simulink model "model_aggressive"  (R2021a)
settings: Solver=VariableStepAuto  StartTime=0.0  StopTime=ToA(end)  RelTol=1e-3
values from neighbouring files (symbols this model uses):
  I = [Jx Jxy Jxz ... (first row only)    [init.m]
  m = 1.5    [init.m]
  pos_ref = [ pos_refx' pos_refy' pos_refz' ]    [trajplann3.m]
  t_ref = []    [trajplann3.m]
  vel_ref = [ vel_refx, vel_refy, vel_refz ]    [trajplann3.m]
undefined symbols (not defined in the file or in its folder): psi
libraries: pid_lib x6, vrlib x4, simulink x1
settings Model: Creator=iris  LastModifiedBy=iris

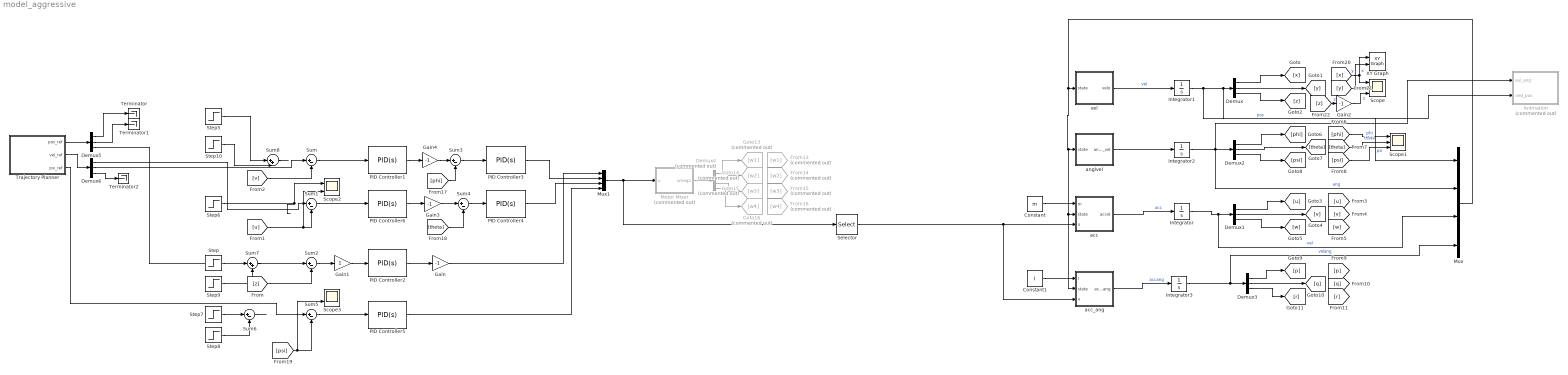
== system model_aggressive ==
  Animation : Subsystem  Commented=on
  Constant : Constant  Value=m
  Constant1 : Constant  Value=I
  Demux{,1..3,5..6} (6 alike) : Demux  Outputs=3
  Demux4 : Demux  Commented=on
  From13 : From  Commented=on  GotoTag=w1
  From14 : From  Commented=on  GotoTag=w2
  From15 : From  Commented=on  GotoTag=w3
  From16 : From  Commented=on  GotoTag=w4
  Gain{,2..4} (4 alike) : Gain  Gain=-1
  Gain1 : Gain
  Goto13 : Goto  Commented=on  GotoTag=w1
  Goto14 : Goto  Commented=on  GotoTag=w2
  Goto15 : Goto  Commented=on  GotoTag=w3
  Goto16 : Goto  Commented=on  GotoTag=w4
  Integrator{,1..3} (4 alike) : Integrator  InitialCondition=[0,0,0]
  Motor Mixer : MATLAB Function  Commented=on  TreatAsAtomicUnit=on
  Mux : Mux
  Mux1 : Mux
  PID Controller1 : pid_lib/PID Controller  Controller=PID  Form=Parallel  TimeDomain=Continuous-time  UseExternalTs=off  SampleTime=-1  IntegratorMethod=Forward Euler  FilterMethod=Forward Euler  ControllerParametersSource=internal  P=0.15  I=0  D=0.009  UseFilter=on  N=100  TunerSelectOption=Transfer Function Based (PID Tuner App)  InitialConditionSource=internal  InitialConditionForIntegrator=0  InitialConditionForFilter=0  DifferentiatorICPrevScaledInput=0  ExternalReset=none  TrackingMode=off  Kt=1  LimitOutput=off  SatLimitsSource=internal  UpperSaturationLimit=inf  LowerSaturationLimit=-inf  LinearizeAsGain=on  AntiWindupMode=none  Kb=1  POutMin=[]  POutMax=[]  IOutMin=[]  IOutMax=[]  DOutMin=[]  DOutMax=[]  NOutMin=[]  NOutMax=[]  SumOutMin=[]  SumOutMax=[]  SaturationOutMin=[]  SaturationOutMax=[]  PParamMin=[]  PParamMax=[]  IParamMin=[]  IParamMax=[]  DParamMin=[]  DParamMax=[]  NParamMin=[]  NParamMax=[]  KbParamMin=[]  KbParamMax=[]  KtParamMin=[]  KtParamMax=[]  KbOutMin=[]  KbOutMax=[]  KtOutMin=[]  KtOutMax=[]  IntegratorOutMin=[]  IntegratorOutMax=[]  FilterOutMin=[]  FilterOutMax=[]  SumI1OutMin=[]  SumI1OutMax=[]  SumI2OutMin=[]  SumI2OutMax=[]  SumI3OutMin=[]  SumI3OutMax=[]  SumI4OutMin=[]  SumI4OutMax=[]  SumDOutMin=[]  SumDOutMax=[]  DifferentiatorOutMin=[]  DifferentiatorOutMax=[]  FilterDiffOutCoefMin=[]  FilterDiffOutCoefMax=[]  ReciprocalOutMin=[]  ReciprocalOutMax=[]  SumDenOutMin=[]  SumDenOutMax=[]  SumNumOutMin=[]  SumNumOutMax=[]  DivideOutMin=[]  DivideOutMax=[]  UdiffTsProdOutMin=[]  UdiffTsProdOutMax=[]  NTsProdOutMin=[]  NTsProdOutMax=[]  UintegralTsProdOutMin=[]  UintegralTsProdOutMax=[]  UngainTsProdOutMin=[]  UngainTsProdOutMax=[]  IntegratorContinuousStateAttributes=''  IntegratorStateMustResolveToSignalObject=off  IntegratorRTWStateStorageClass=Auto  FilterContinuousStateAttributes=''  FilterStateMustResolveToSignalObject=off  FilterRTWStateStorageClass=Auto  ParallelPVariant=InternalParameters  IdealPVariant=Disabled  IVariant=InternalParameters  DVariant=InternalParameters  IntegratorVariant=Continuous  SatVariant=Disabled  AWVariant=Passthrough  PCopyVariant=Disabled  TRVariant=Disabled  FdbkBlocksVariant=Forward  IdealPFdbkVariant=Disabled  SatFdbkVariant=Disabled  DerivativeFilterVariant=ContFilter  NVariant=InternalParameters  NCopyVariant=Disabled  FilterICVariant=InternalICsFilter  IntegratorICVariant=InternalICs  ExternalResetVariant=Disabled  TRSumVariant=Passthrough  SumFdbkVariant=Disabled  SumVariant=Sum_PID  TsampFilterVariant=InternalTs  TsampNgainVariant=Passthrough  TsampIntegralVariant=Passthrough  ExternalSaturationOutDataTypeStr=Inherit: Same as second input
  PID Controller2 : pid_lib/PID Controller  Controller=PID  Form=Parallel  TimeDomain=Continuous-time  UseExternalTs=off  SampleTime=-1  IntegratorMethod=Forward Euler  FilterMethod=Forward Euler  ControllerParametersSource=internal  P=60  I=70  D=40  UseFilter=on  N=100  TunerSelectOption=Transfer Function Based (PID Tuner App)  InitialConditionSource=internal  InitialConditionForIntegrator=0  InitialConditionForFilter=0  DifferentiatorICPrevScaledInput=0  ExternalReset=none  TrackingMode=off  Kt=1  LimitOutput=off  SatLimitsSource=internal  UpperSaturationLimit=inf  LowerSaturationLimit=-inf  LinearizeAsGain=on  AntiWindupMode=none  Kb=1  POutMin=[]  POutMax=[]  IOutMin=[]  IOutMax=[]  DOutMin=[]  DOutMax=[]  NOutMin=[]  NOutMax=[]  SumOutMin=[]  SumOutMax=[]  SaturationOutMin=[]  SaturationOutMax=[]  PParamMin=[]  PParamMax=[]  IParamMin=[]  IParamMax=[]  DParamMin=[]  DParamMax=[]  NParamMin=[]  NParamMax=[]  KbParamMin=[]  KbParamMax=[]  KtParamMin=[]  KtParamMax=[]  KbOutMin=[]  KbOutMax=[]  KtOutMin=[]  KtOutMax=[]  IntegratorOutMin=[]  IntegratorOutMax=[]  FilterOutMin=[]  FilterOutMax=[]  SumI1OutMin=[]  SumI1OutMax=[]  SumI2OutMin=[]  SumI2OutMax=[]  SumI3OutMin=[]  SumI3OutMax=[]  SumI4OutMin=[]  SumI4OutMax=[]  SumDOutMin=[]  SumDOutMax=[]  DifferentiatorOutMin=[]  DifferentiatorOutMax=[]  FilterDiffOutCoefMin=[]  FilterDiffOutCoefMax=[]  ReciprocalOutMin=[]  ReciprocalOutMax=[]  SumDenOutMin=[]  SumDenOutMax=[]  SumNumOutMin=[]  SumNumOutMax=[]  DivideOutMin=[]  DivideOutMax=[]  UdiffTsProdOutMin=[]  UdiffTsProdOutMax=[]  NTsProdOutMin=[]  NTsProdOutMax=[]  UintegralTsProdOutMin=[]  UintegralTsProdOutMax=[]  UngainTsProdOutMin=[]  UngainTsProdOutMax=[]  IntegratorContinuousStateAttributes=''  IntegratorStateMustResolveToSignalObject=off  IntegratorRTWStateStorageClass=Auto  FilterContinuousStateAttributes=''  FilterStateMustResolveToSignalObject=off  FilterRTWStateStorageClass=Auto  ParallelPVariant=InternalParameters  IdealPVariant=Disabled  IVariant=InternalParameters  DVariant=InternalParameters  IntegratorVariant=Continuous  SatVariant=Disabled  AWVariant=Passthrough  PCopyVariant=Disabled  TRVariant=Disabled  FdbkBlocksVariant=Forward  IdealPFdbkVariant=Disabled  SatFdbkVariant=Disabled  DerivativeFilterVariant=ContFilter  NVariant=InternalParameters  NCopyVariant=Disabled  FilterICVariant=InternalICsFilter  IntegratorICVariant=InternalICs  ExternalResetVariant=Disabled  TRSumVariant=Passthrough  SumFdbkVariant=Disabled  SumVariant=Sum_PID  TsampFilterVariant=InternalTs  TsampNgainVariant=Passthrough  TsampIntegralVariant=Passthrough  ExternalSaturationOutDataTypeStr=Inherit: Same as second input
  PID Controller3 : pid_lib/PID Controller  Controller=PID  Form=Parallel  TimeDomain=Continuous-time  UseExternalTs=off  SampleTime=-1  IntegratorMethod=Forward Euler  FilterMethod=Forward Euler  ControllerParametersSource=internal  P=0.08  I=0.02  D=0.08  UseFilter=on  N=100  TunerSelectOption=Transfer Function Based (PID Tuner App)  InitialConditionSource=internal  InitialConditionForIntegrator=0  InitialConditionForFilter=0  DifferentiatorICPrevScaledInput=0  ExternalReset=none  TrackingMode=off  Kt=1  LimitOutput=off  SatLimitsSource=internal  UpperSaturationLimit=inf  LowerSaturationLimit=-inf  LinearizeAsGain=on  AntiWindupMode=none  Kb=1  POutMin=[]  POutMax=[]  IOutMin=[]  IOutMax=[]  DOutMin=[]  DOutMax=[]  NOutMin=[]  NOutMax=[]  SumOutMin=[]  SumOutMax=[]  SaturationOutMin=[]  SaturationOutMax=[]  PParamMin=[]  PParamMax=[]  IParamMin=[]  IParamMax=[]  DParamMin=[]  DParamMax=[]  NParamMin=[]  NParamMax=[]  KbParamMin=[]  KbParamMax=[]  KtParamMin=[]  KtParamMax=[]  KbOutMin=[]  KbOutMax=[]  KtOutMin=[]  KtOutMax=[]  IntegratorOutMin=[]  IntegratorOutMax=[]  FilterOutMin=[]  FilterOutMax=[]  SumI1OutMin=[]  SumI1OutMax=[]  SumI2OutMin=[]  SumI2OutMax=[]  SumI3OutMin=[]  SumI3OutMax=[]  SumI4OutMin=[]  SumI4OutMax=[]  SumDOutMin=[]  SumDOutMax=[]  DifferentiatorOutMin=[]  DifferentiatorOutMax=[]  FilterDiffOutCoefMin=[]  FilterDiffOutCoefMax=[]  ReciprocalOutMin=[]  ReciprocalOutMax=[]  SumDenOutMin=[]  SumDenOutMax=[]  SumNumOutMin=[]  SumNumOutMax=[]  DivideOutMin=[]  DivideOutMax=[]  UdiffTsProdOutMin=[]  UdiffTsProdOutMax=[]  NTsProdOutMin=[]  NTsProdOutMax=[]  UintegralTsProdOutMin=[]  UintegralTsProdOutMax=[]  UngainTsProdOutMin=[]  UngainTsProdOutMax=[]  IntegratorContinuousStateAttributes=''  IntegratorStateMustResolveToSignalObject=off  IntegratorRTWStateStorageClass=Auto  FilterContinuousStateAttributes=''  FilterStateMustResolveToSignalObject=off  FilterRTWStateStorageClass=Auto  ParallelPVariant=InternalParameters  IdealPVariant=Disabled  IVariant=InternalParameters  DVariant=InternalParameters  IntegratorVariant=Continuous  SatVariant=Disabled  AWVariant=Passthrough  PCopyVariant=Disabled  TRVariant=Disabled  FdbkBlocksVariant=Forward  IdealPFdbkVariant=Disabled  SatFdbkVariant=Disabled  DerivativeFilterVariant=ContFilter  NVariant=InternalParameters  NCopyVariant=Disabled  FilterICVariant=InternalICsFilter  IntegratorICVariant=InternalICs  ExternalResetVariant=Disabled  TRSumVariant=Passthrough  SumFdbkVariant=Disabled  SumVariant=Sum_PID  TsampFilterVariant=InternalTs  TsampNgainVariant=Passthrough  TsampIntegralVariant=Passthrough  ExternalSaturationOutDataTypeStr=Inherit: Same as second input
  PID Controller4 : pid_lib/PID Controller  Controller=PID  Form=Parallel  TimeDomain=Continuous-time  UseExternalTs=off  SampleTime=-1  IntegratorMethod=Forward Euler  FilterMethod=Forward Euler  ControllerParametersSource=internal  P=0.08  I=0.02  D=0.08  UseFilter=on  N=100  TunerSelectOption=Transfer Function Based (PID Tuner App)  InitialConditionSource=internal  InitialConditionForIntegrator=0  InitialConditionForFilter=0  DifferentiatorICPrevScaledInput=0  ExternalReset=none  TrackingMode=off  Kt=1  LimitOutput=off  SatLimitsSource=internal  UpperSaturationLimit=inf  LowerSaturationLimit=-inf  LinearizeAsGain=on  AntiWindupMode=none  Kb=1  POutMin=[]  POutMax=[]  IOutMin=[]  IOutMax=[]  DOutMin=[]  DOutMax=[]  NOutMin=[]  NOutMax=[]  SumOutMin=[]  SumOutMax=[]  SaturationOutMin=[]  SaturationOutMax=[]  PParamMin=[]  PParamMax=[]  IParamMin=[]  IParamMax=[]  DParamMin=[]  DParamMax=[]  NParamMin=[]  NParamMax=[]  KbParamMin=[]  KbParamMax=[]  KtParamMin=[]  KtParamMax=[]  KbOutMin=[]  KbOutMax=[]  KtOutMin=[]  KtOutMax=[]  IntegratorOutMin=[]  IntegratorOutMax=[]  FilterOutMin=[]  FilterOutMax=[]  SumI1OutMin=[]  SumI1OutMax=[]  SumI2OutMin=[]  SumI2OutMax=[]  SumI3OutMin=[]  SumI3OutMax=[]  SumI4OutMin=[]  SumI4OutMax=[]  SumDOutMin=[]  SumDOutMax=[]  DifferentiatorOutMin=[]  DifferentiatorOutMax=[]  FilterDiffOutCoefMin=[]  FilterDiffOutCoefMax=[]  ReciprocalOutMin=[]  ReciprocalOutMax=[]  SumDenOutMin=[]  SumDenOutMax=[]  SumNumOutMin=[]  SumNumOutMax=[]  DivideOutMin=[]  DivideOutMax=[]  UdiffTsProdOutMin=[]  UdiffTsProdOutMax=[]  NTsProdOutMin=[]  NTsProdOutMax=[]  UintegralTsProdOutMin=[]  UintegralTsProdOutMax=[]  UngainTsProdOutMin=[]  UngainTsProdOutMax=[]  IntegratorContinuousStateAttributes=''  IntegratorStateMustResolveToSignalObject=off  IntegratorRTWStateStorageClass=Auto  FilterContinuousStateAttributes=''  FilterStateMustResolveToSignalObject=off  FilterRTWStateStorageClass=Auto  ParallelPVariant=InternalParameters  IdealPVariant=Disabled  IVariant=InternalParameters  DVariant=InternalParameters  IntegratorVariant=Continuous  SatVariant=Disabled  AWVariant=Passthrough  PCopyVariant=Disabled  TRVariant=Disabled  FdbkBlocksVariant=Forward  IdealPFdbkVariant=Disabled  SatFdbkVariant=Disabled  DerivativeFilterVariant=ContFilter  NVariant=InternalParameters  NCopyVariant=Disabled  FilterICVariant=InternalICsFilter  IntegratorICVariant=InternalICs  ExternalResetVariant=Disabled  TRSumVariant=Passthrough  SumFdbkVariant=Disabled  SumVariant=Sum_PID  TsampFilterVariant=InternalTs  TsampNgainVariant=Passthrough  TsampIntegralVariant=Passthrough  ExternalSaturationOutDataTypeStr=Inherit: Same as second input
  PID Controller5 : pid_lib/PID Controller  Controller=PID  Form=Parallel  TimeDomain=Continuous-time  UseExternalTs=off  SampleTime=-1  IntegratorMethod=Forward Euler  FilterMethod=Forward Euler  ControllerParametersSource=internal  P=0.15  I=0.0001  D=0.2  UseFilter=on  N=100  TunerSelectOption=Transfer Function Based (PID Tuner App)  InitialConditionSource=internal  InitialConditionForIntegrator=0  InitialConditionForFilter=0  DifferentiatorICPrevScaledInput=0  ExternalReset=none  TrackingMode=off  Kt=1  LimitOutput=off  SatLimitsSource=internal  UpperSaturationLimit=inf  LowerSaturationLimit=-inf  LinearizeAsGain=on  AntiWindupMode=none  Kb=1  POutMin=[]  POutMax=[]  IOutMin=[]  IOutMax=[]  DOutMin=[]  DOutMax=[]  NOutMin=[]  NOutMax=[]  SumOutMin=[]  SumOutMax=[]  SaturationOutMin=[]  SaturationOutMax=[]  PParamMin=[]  PParamMax=[]  IParamMin=[]  IParamMax=[]  DParamMin=[]  DParamMax=[]  NParamMin=[]  NParamMax=[]  KbParamMin=[]  KbParamMax=[]  KtParamMin=[]  KtParamMax=[]  KbOutMin=[]  KbOutMax=[]  KtOutMin=[]  KtOutMax=[]  IntegratorOutMin=[]  IntegratorOutMax=[]  FilterOutMin=[]  FilterOutMax=[]  SumI1OutMin=[]  SumI1OutMax=[]  SumI2OutMin=[]  SumI2OutMax=[]  SumI3OutMin=[]  SumI3OutMax=[]  SumI4OutMin=[]  SumI4OutMax=[]  SumDOutMin=[]  SumDOutMax=[]  DifferentiatorOutMin=[]  DifferentiatorOutMax=[]  FilterDiffOutCoefMin=[]  FilterDiffOutCoefMax=[]  ReciprocalOutMin=[]  ReciprocalOutMax=[]  SumDenOutMin=[]  SumDenOutMax=[]  SumNumOutMin=[]  SumNumOutMax=[]  DivideOutMin=[]  DivideOutMax=[]  UdiffTsProdOutMin=[]  UdiffTsProdOutMax=[]  NTsProdOutMin=[]  NTsProdOutMax=[]  UintegralTsProdOutMin=[]  UintegralTsProdOutMax=[]  UngainTsProdOutMin=[]  UngainTsProdOutMax=[]  IntegratorContinuousStateAttributes=''  IntegratorStateMustResolveToSignalObject=off  IntegratorRTWStateStorageClass=Auto  FilterContinuousStateAttributes=''  FilterStateMustResolveToSignalObject=off  FilterRTWStateStorageClass=Auto  ParallelPVariant=InternalParameters  IdealPVariant=Disabled  IVariant=InternalParameters  DVariant=InternalParameters  IntegratorVariant=Continuous  SatVariant=Disabled  AWVariant=Passthrough  PCopyVariant=Disabled  TRVariant=Disabled  FdbkBlocksVariant=Forward  IdealPFdbkVariant=Disabled  SatFdbkVariant=Disabled  DerivativeFilterVariant=ContFilter  NVariant=InternalParameters  NCopyVariant=Disabled  FilterICVariant=InternalICsFilter  IntegratorICVariant=InternalICs  ExternalResetVariant=Disabled  TRSumVariant=Passthrough  SumFdbkVariant=Disabled  SumVariant=Sum_PID  TsampFilterVariant=InternalTs  TsampNgainVariant=Passthrough  TsampIntegralVariant=Passthrough  ExternalSaturationOutDataTypeStr=Inherit: Same as second input
  PID Controller6 : pid_lib/PID Controller  Controller=PID  Form=Parallel  TimeDomain=Continuous-time  UseExternalTs=off  SampleTime=-1  IntegratorMethod=Forward Euler  FilterMethod=Forward Euler  ControllerParametersSource=internal  P=0.15  I=0  D=0.009  UseFilter=on  N=100  TunerSelectOption=Transfer Function Based (PID Tuner App)  InitialConditionSource=internal  InitialConditionForIntegrator=0  InitialConditionForFilter=0  DifferentiatorICPrevScaledInput=0  ExternalReset=none  TrackingMode=off  Kt=1  LimitOutput=off  SatLimitsSource=internal  UpperSaturationLimit=inf  LowerSaturationLimit=-inf  LinearizeAsGain=on  AntiWindupMode=none  Kb=1  POutMin=[]  POutMax=[]  IOutMin=[]  IOutMax=[]  DOutMin=[]  DOutMax=[]  NOutMin=[]  NOutMax=[]  SumOutMin=[]  SumOutMax=[]  SaturationOutMin=[]  SaturationOutMax=[]  PParamMin=[]  PParamMax=[]  IParamMin=[]  IParamMax=[]  DParamMin=[]  DParamMax=[]  NParamMin=[]  NParamMax=[]  KbParamMin=[]  KbParamMax=[]  KtParamMin=[]  KtParamMax=[]  KbOutMin=[]  KbOutMax=[]  KtOutMin=[]  KtOutMax=[]  IntegratorOutMin=[]  IntegratorOutMax=[]  FilterOutMin=[]  FilterOutMax=[]  SumI1OutMin=[]  SumI1OutMax=[]  SumI2OutMin=[]  SumI2OutMax=[]  SumI3OutMin=[]  SumI3OutMax=[]  SumI4OutMin=[]  SumI4OutMax=[]  SumDOutMin=[]  SumDOutMax=[]  DifferentiatorOutMin=[]  DifferentiatorOutMax=[]  FilterDiffOutCoefMin=[]  FilterDiffOutCoefMax=[]  ReciprocalOutMin=[]  ReciprocalOutMax=[]  SumDenOutMin=[]  SumDenOutMax=[]  SumNumOutMin=[]  SumNumOutMax=[]  DivideOutMin=[]  DivideOutMax=[]  UdiffTsProdOutMin=[]  UdiffTsProdOutMax=[]  NTsProdOutMin=[]  NTsProdOutMax=[]  UintegralTsProdOutMin=[]  UintegralTsProdOutMax=[]  UngainTsProdOutMin=[]  UngainTsProdOutMax=[]  IntegratorContinuousStateAttributes=''  IntegratorStateMustResolveToSignalObject=off  IntegratorRTWStateStorageClass=Auto  FilterContinuousStateAttributes=''  FilterStateMustResolveToSignalObject=off  FilterRTWStateStorageClass=Auto  ParallelPVariant=InternalParameters  IdealPVariant=Disabled  IVariant=InternalParameters  DVariant=InternalParameters  IntegratorVariant=Continuous  SatVariant=Disabled  AWVariant=Passthrough  PCopyVariant=Disabled  TRVariant=Disabled  FdbkBlocksVariant=Forward  IdealPFdbkVariant=Disabled  SatFdbkVariant=Disabled  DerivativeFilterVariant=ContFilter  NVariant=InternalParameters  NCopyVariant=Disabled  FilterICVariant=InternalICsFilter  IntegratorICVariant=InternalICs  ExternalResetVariant=Disabled  TRSumVariant=Passthrough  SumFdbkVariant=Disabled  SumVariant=Sum_PID  TsampFilterVariant=InternalTs  TsampNgainVariant=Passthrough  TsampIntegralVariant=Passthrough  ExternalSaturationOutDataTypeStr=Inherit: Same as second input
  Scope : Scope  NumInputPorts=3
  Scope1 : Scope  NumInputPorts=3
  Scope2 : Scope  NumInputPorts=2
  Scope3 : Scope  NumInputPorts=2
  Selector : Selector  InputPortWidth=4  IndexOptions=Index vector (dialog)  Indices=[1 2 3 4]  OutputSizes=1
  Step : Step  After=-2  SampleTime=0
  Step10 : Step  Time=9  After=-0.5  SampleTime=0
  Step5 : Step  Time=2  After=0.5  SampleTime=0
  Step6 : Step  Time=3  After=0  SampleTime=0
  Step7 : Step  After=0  SampleTime=0
  Step8 : Step  Time=9  After=0  SampleTime=0
  Step9 : Step  Time=9  After=2  SampleTime=0
  Sum{,1..6} (7 alike) : Sum  Inputs=|+-
  Sum7 : Sum  Inputs=|++
  Sum8 : Sum  Inputs=|++
  Terminator : Terminator
  Terminator1 : Terminator
  Terminator2 : Terminator
  Trajectory Planner : Subsystem
  XY Graph : simulink/Sinks/XY Graph  xmin=-10  xmax=10  ymin=-10  ymax=10  st=-1
  acc : MATLAB Function  TreatAsAtomicUnit=on
  acc_ang : MATLAB Function  TreatAsAtomicUnit=on
  anglvel : MATLAB Function  TreatAsAtomicUnit=on
  vel : MATLAB Function  TreatAsAtomicUnit=on
  wires:
  Constant/1 -> acc/1(m)
  Constant1/1 -> acc_ang/1(I)
  Motor Mixer/1(omega) -> Demux4/1
  Demux4/1 -> Goto13/1
  Demux4/2 -> Goto14/1
  Demux4/3 -> Goto15/1
  Demux4/4 -> Goto16/1
  [v] -> Sum/2
  [u] -> Scope2/2, Sum1/2
  [z] -> Sum2/2
  Sum2/1 -> Gain1/1
  Sum1/1 -> PID Controller6/1
  Sum/1 -> PID Controller1/1
  Sum3/1 -> PID Controller3/1
  [phi] -> Sum3/2
  Sum4/1 -> PID Controller4/1
  [theta] -> Sum4/2
  PID Controller6/1 -> Gain3/1
  PID Controller1/1 -> Gain4/1
  Sum5/1 -> PID Controller5/1
  [psi] -> Scope3/2, Sum5/2
  PID Controller3/1 -> Mux1/2
  PID Controller4/1 -> Mux1/3
  PID Controller2/1 -> Gain/1
  PID Controller5/1 -> Mux1/4
  Mux1/1 -> Selector/1, Motor Mixer/1(u)
  Integrator3/1 -> Mux/4, Demux3/1  "velang"
  Demux/3 -> [z]
  Integrator/1 -> Mux/3, Demux1/1  "vel"
  Demux3/3 -> [r]
  Integrator2/1 -> Animation/1(eul_ang), Demux2/1, Mux/2  "ang"
  acc_ang/1(accel_ang) -> Integrator3/1  "accang"
  Demux/1 -> [x]
  Demux2/1 -> [phi]
  Demux2/3 -> [psi]
  Demux1/3 -> [w]
  Demux3/1 -> [p]
  anglvel/1(angular_vel) -> Integrator2/1
  Integrator1/1 -> Animation/2(ned_pos), Mux/1, Demux/1  "pos"
  Demux1/1 -> [u]
  Demux3/2 -> [q]
  Demux/2 -> [y]
  Demux1/2 -> [v]
  Demux2/2 -> [theta]
  acc/1(accel) -> Integrator/1  "acc"
  vel/1(velo) -> Integrator1/1  "vel"
  Mux/1 -> acc_ang/2(state), acc/2(state), anglvel/1(state), vel/1(state)
  [x] -> XY Graph/1, Scope/1  "x"
  [y] -> Scope/2, XY Graph/2  "y"
  [z] -> Gain2/1  "z"
  Selector/1 -> acc/3(u), acc_ang/3(u)
  Gain/1 -> Mux1/1
  Gain1/1 -> PID Controller2/1
  Gain2/1 -> Scope/3  "z"
  [phi] -> Scope1/1  "phi"
  [theta] -> Scope1/2  "theta"
  [psi] -> Scope1/3  "psi"
  Gain3/1 -> Sum4/1
  Gain4/1 -> Sum3/1
  Step6/1 -> Scope2/1
  Step/1 -> Sum7/1
  Step5/1 -> Sum8/1
  Step7/1 -> Sum6/1
  Step8/1 -> Sum6/2
  Sum6/1 -> ?
  Sum7/1 -> ?
  Step9/1 -> Sum7/2
  Step10/1 -> Sum8/2
  Sum8/1 -> ?
  Trajectory Planner/1(pos_ref) -> Demux5/1
  Demux5/1 -> Terminator/1
  Demux5/2 -> Terminator1/1
  Demux5/3 -> Sum2/1
  Trajectory Planner/2(vel_ref) -> Demux6/1
  Demux6/1 -> Sum1/1
  Demux6/2 -> Sum/1
  Demux6/3 -> Terminator2/1
  Trajectory Planner/3(psi_ref) -> Sum5/1

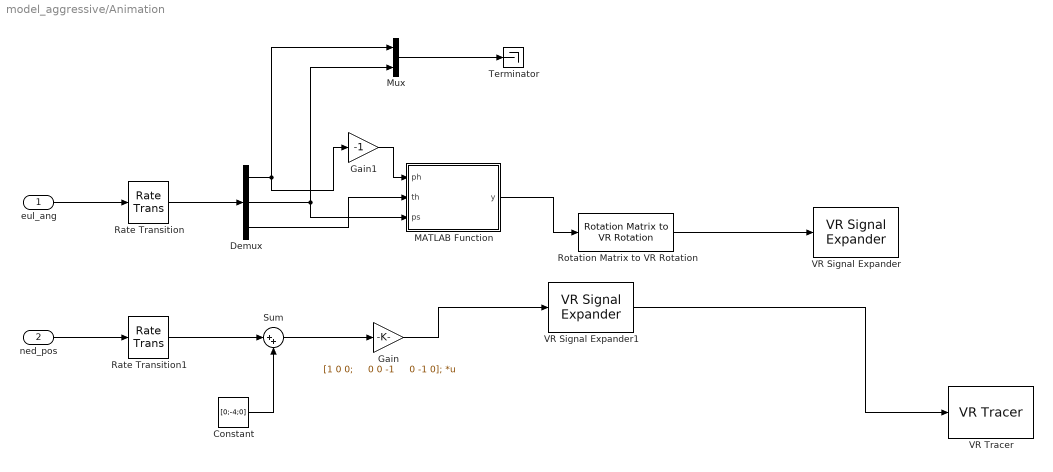
== system model_aggressive/Animation ==
  eul_ang : Inport
  ned_pos : Inport  Port=2
  Constant : Constant  Value=[0;-4;0]
  Demux : Demux  Outputs=3
  Gain : Gain  Gain=|  Multiplication=Matrix(K*u)
      | [1 0 0;
      |     0 0 -1
      |     0 -1 0];
  Gain1 : Gain  Gain=-1
  MATLAB Function : MATLAB Function  TreatAsAtomicUnit=on
  Mux : Mux  Inputs=2
  Rate Transition : RateTransition  OutPortSampleTime=0.1
  Rate Transition1 : RateTransition  OutPortSampleTime=0.1
  Rotation Matrix to VR Rotation : vrlib/Utilities/Rotation Matrix to VR Rotation  maxzero=1e-12
      settings: SourceProductBaseCode=SL
  Sum : Sum  Inputs=|++
  Terminator : Terminator
  VR Signal Expander : vrlib/VR Signal Expander  outwidth=4  outidx=[1:4]
  VR Signal Expander1 : vrlib/VR Signal Expander  outwidth=3  outidx=[1:3]
  VR Tracer : vrlib/VR Tracer  VrmlFile=uav_scene.x3dv  MarkerName=Sphere  UseLines=on  UseTriads=on  MarkerScale=[0.1 0.1 0.1]  MarkerColorSelection=Selected from color list  MarkerColor=red  rgbval=[1 0 0]  Ts=0.5  ForceViewerOpen=off  ConnectPlane=off  PlaneCoeff=[0 1 0 0]  ConnectPoint=None  PointCoord=[0 0 0]
      settings: SourceProductBaseCode=SL
  wires:
  ned_pos/1 -> Rate Transition1/1
  eul_ang/1 -> Rate Transition/1
  Demux/1 -> Gain1/1, Mux/1
  Rotation Matrix to VR Rotation/1 -> VR Signal Expander/1
  Rate Transition1/1 -> Sum/1
  Rate Transition/1 -> Demux/1
  Mux/1 -> Terminator/1
  VR Signal Expander1/1 -> VR Tracer/1
  Gain/1 -> VR Signal Expander1/1
  MATLAB Function/1(y) -> Rotation Matrix to VR Rotation/1
  Demux/3 -> MATLAB Function/2(th)
  Demux/2 -> MATLAB Function/3(ps), Mux/2
  Gain1/1 -> MATLAB Function/1(ph)
  Sum/1 -> Gain/1
  Constant/1 -> Sum/2

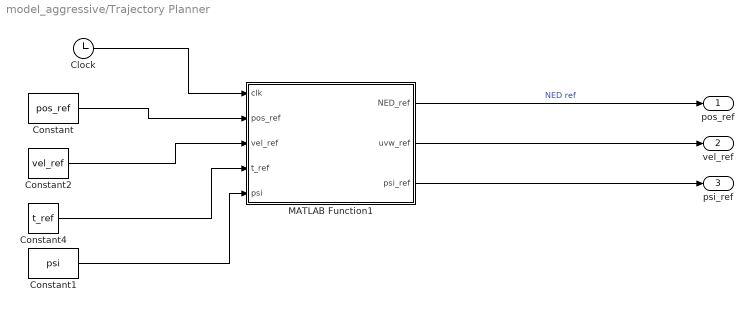
== system model_aggressive/Trajectory Planner ==
  Clock : Clock
  Constant : Constant  Value=pos_ref
  Constant1 : Constant  Value=psi
  Constant2 : Constant  Value=vel_ref
  Constant4 : Constant  Value=t_ref
  MATLAB Function1 : MATLAB Function  TreatAsAtomicUnit=on
  pos_ref : Outport
  vel_ref : Outport  Port=2
  psi_ref : Outport  Port=3
  wires:
  Constant/1 -> MATLAB Function1/2(pos_ref)
  Constant2/1 -> MATLAB Function1/3(vel_ref)
  Constant4/1 -> MATLAB Function1/4(t_ref)
  Clock/1 -> MATLAB Function1/1(clk)
  Constant1/1 -> MATLAB Function1/5(psi)
  MATLAB Function1/1(NED_ref) -> pos_ref/1  "NED ref"
  MATLAB Function1/2(uvw_ref) -> vel_ref/1
  MATLAB Function1/3(psi_ref) -> psi_ref/1

== matlab function model_aggressive/vel ==
  data: state input; velo output
function velo = vel(state)

ph = state(4);
th = state(5);
ps = state(6);

Rot_mat = [cos(th)*cos(ps) sin(ph)*sin(th)*cos(ps)-cos(ph)*sin(ps) cos(ph)*sin(th)*cos(ps)+sin(ph)*sin(ps);
    cos(th)*sin(ps) sin(ph)*sin(th)*sin(ps)+cos(ph)*cos(ps) cos(ph)*sin(th)*sin(ps)-sin(ph)*cos(ps);
    -sin(th) sin(ph)*cos(th) cos(ph)*cos(th)]; % body to NED

velo = Rot_mat*state(7:9);
% xdot = velo(1);
% ydot = velo(2);
% zdot = velo(3);

== matlab function model_aggressive/acc ==
  data: m input; state input; u input; accel output
function accel = acc(m,state,u)


ph = state(4);
th = state(5);
ps = state(6);
udot = -1/m*(cos(ph)*sin(th)*cos(ps)+sin(ph)*sin(ps))*u(1);
vdot = -1/m*(cos(ph)*sin(th)*sin(ps)+sin(ph)*cos(ps))*u(1);
wdot = 9.81 - 1/m*(cos(ph)*cos(th))*u(1);

accel = [udot
         vdot
         wdot];

== matlab function model_aggressive/anglvel ==
  data: state input; angular_vel output
function angular_vel = angvel(state)

ph = state(4);
th = state(5);
ps = state(6);
p = state(10);
q = state(11);
r = state(12);

phi_dot = p + (sin(ph)*tan(th))*q - (cos(ph)*tan(th))*r;
theta_dot = cos(ph)*q + sin(ph)*r;
psi_dot = -1*(sin(ph)*sec(th)*q) + (cos(ph)*sec(th))*r;


% angular_vel(1) = phi_dot;
% angular_vel(2) = theta_dot;
% angular_vel(3) = psi_dot;
angular_vel = [phi_dot,theta_dot,psi_dot];

== matlab function model_aggressive/acc_ang ==
  data: I input; state input; u input; accel_ang output
function accel_ang = acc_ang(I,state,u)

p = state(10);
q = state(11);
r = state(12);
T = u(1);
tau_x = u(2,1);
tau_y = u(3,1);
tau_z = u(4,1);

Ix = I(1,1);
Iy = I(2,2);
Iz = I(3,3);
Ixy = I(1,2);
Ixz = I(1,3);
Iyz = I(2,3);

pdot = (Iy-Iz)/Ix*q*r + 1/Ix*tau_x;
qdot = (Iz-Ix)/Iy*p*r + 1/Iy*tau_y;
rdot = (Ix-Iy)/Iz*p*q + 1/Iz*tau_z;


accel_ang = [pdot
             qdot
             rdot];

== matlab function model_aggressive/Motor Mixer ==
  data: u input; omega output
function omega = mixer(u)

k = 1;
l = 0.25;
b = 1;

mat = [k k k k;
      0 l*k 0 -l*k;
      l*k 0 -l*k 0;
      b -b b -b];
  
om = u\mat;
omega = sqrt(om);

== matlab function model_aggressive/Animation/MATLAB Function ==
  data: ph input; y output; th input; ps input
function y = fcn(ph,th,ps)

Rb_ned = [ cos(th)*cos(ps), cos(th)*sin(ps), -sin(th)
            -cos(ph)*sin(ps) + sin(ph)*sin(th)*cos(ps), cos(ph)...
                *cos(ps) + sin(ph)*sin(th)*sin(ps), sin(ph)*cos(th)
            sin(ph)*sin(ps) + cos(ph)*sin(th)*cos(ps), -sin(ph)...
            *cos(ps) + cos(ph)*sin(th)*sin(ps), cos(ph)*cos(th) ];
Rx = [1 0 0;
    0 1 0
    0 0 1];
        
y = Rx*Rb_ned';

== matlab function model_aggressive/Trajectory Planner/MATLAB Function1 ==
  data: clk input; NED_ref output; pos_ref input; vel_ref input; t_ref input; uvw_ref output; psi_ref output; psi input
function [ NED_ref, uvw_ref, psi_ref]  = trajectoryPlanner(clk,pos_ref,vel_ref,t_ref,psi)

currTime = find(clk >= t_ref);
NED_ref = pos_ref(currTime(end),:)';
uvw_ref = vel_ref(currTime(end),:)';
psi_ref = psi(currTime(end),:)';

end
